simulink model "Final_V620140905h5b_fuben1"  (Simulink 7.9)
settings: Solver=FixedStepDiscrete  StartTime=0.0  StopTime=1  FixedStep=Auto  RelTol=1e-3
undefined symbols (not defined in the file or in its folder): Down, Up
libraries: tiiqmathlib x157, idelinklib_common x83, c2833xlib x37, simulink x12, c28xdmclib x12, c280xlib x7, simulink_extras x4, commutil2 x2, idelinklib_tgtpref x1, idelinklib_ticcs x1
(part 6 of 7)

== system Final_V620140905h5b_fuben1/Function-Call Subsystem1/AD/Read AD ==
  note: M2
  note: M1
  note: M12
  note: M11
  note: M9
  note: AD1
  note: AD2
  note: M10
  note: M3
  note: M4
  note: M5
  note: M6
  note: M7
  note: M8
  note: IH1
  note: IH3
  note: IH2
  note: IH4
  note: IH5
  note: VH1
  note: VH2
  note: VH9
  Memory Copy1 : idelinklib_common/Memory Copy  Priority=3  copyFrom=Specified address  copyFromAddressSource=Specify via dialog  copyFromAddress=hex2dec('200008')  copyFromSrcCode=myVariableSrc  dataTypeFrom=int16  dataDimensionFrom=1  useOffsetFrom=off  offsetFromSrc=Specify via dialog  offsetFrom=0  strideFrom=1  copyTo=Specified source code symbol  copyToAddressSource=Specify via dialog  copyToAddress=temp  copyToSrcCode=M8  dataTypeTo=int16  useOffsetTo=on  offsetToSrc=Specify via dialog  offsetTo=0  strideTo=1  sampleTime=inf  useInitValue=off  initValueSrc=Specify constant value  initValue=bin2dec('00000000')  initValueSrcCode=myInitValueVariable  useAsMask=off  maskOperator=bitwise AND  useTermValue=off  termValue=bin2dec('00000000')  isRealtimeEnabled=off  emitCCBeforeWrite=off  CCBeforeWrite=/* Custom Code Before Write*/  emitCCAfterWrite=off  CCAfterWrite=/* Custom Code After Write*/  useDMACopy=off  enableBlockingMode=off
  Memory Copy13 : idelinklib_common/Memory Copy  Priority=2  copyFrom=Specified address  copyFromAddressSource=Specify via dialog  copyFromAddress=hex2dec('200008')  copyFromSrcCode=myVariableSrc  dataTypeFrom=int16  dataDimensionFrom=1  useOffsetFrom=off  offsetFromSrc=Specify via dialog  offsetFrom=0  strideFrom=1  copyTo=Specified source code symbol  copyToAddressSource=Specify via dialog  copyToAddress=temp  copyToSrcCode=M7  dataTypeTo=int16  useOffsetTo=on  offsetToSrc=Specify via dialog  offsetTo=0  strideTo=1  sampleTime=inf  useInitValue=off  initValueSrc=Specify constant value  initValue=bin2dec('00000000')  initValueSrcCode=myInitValueVariable  useAsMask=off  maskOperator=bitwise AND  useTermValue=off  termValue=bin2dec('00000000')  isRealtimeEnabled=off  emitCCBeforeWrite=off  CCBeforeWrite=/* Custom Code Before Write*/  emitCCAfterWrite=off  CCAfterWrite=/* Custom Code After Write*/  useDMACopy=off  enableBlockingMode=off
  Memory Copy14 : idelinklib_common/Memory Copy  Priority=12  copyFrom=Specified address  copyFromAddressSource=Specify via dialog  copyFromAddress=hex2dec('200004')  copyFromSrcCode=myVariableSrc  dataTypeFrom=int16  dataDimensionFrom=1  useOffsetFrom=off  offsetFromSrc=Specify via dialog  offsetFrom=0  strideFrom=1  copyTo=Specified source code symbol  copyToAddressSource=Specify via dialog  copyToAddress=temp  copyToSrcCode=M4  dataTypeTo=int16  useOffsetTo=on  offsetToSrc=Specify via dialog  offsetTo=0  strideTo=1  sampleTime=inf  useInitValue=off  initValueSrc=Specify constant value  initValue=bin2dec('00000000')  initValueSrcCode=myInitValueVariable  useAsMask=off  maskOperator=bitwise AND  useTermValue=off  termValue=bin2dec('00000000')  isRealtimeEnabled=off  emitCCBeforeWrite=off  CCBeforeWrite=/* Custom Code Before Write*/  emitCCAfterWrite=off  CCAfterWrite=/* Custom Code After Write*/  useDMACopy=off  enableBlockingMode=off
  Memory Copy15 : idelinklib_common/Memory Copy  Priority=13  copyFrom=Specified address  copyFromAddressSource=Specify via dialog  copyFromAddress=hex2dec('200004')  copyFromSrcCode=myVariableSrc  dataTypeFrom=int16  dataDimensionFrom=1  useOffsetFrom=off  offsetFromSrc=Specify via dialog  offsetFrom=0  strideFrom=1  copyTo=Specified source code symbol  copyToAddressSource=Specify via dialog  copyToAddress=temp  copyToSrcCode=M5  dataTypeTo=int16  useOffsetTo=on  offsetToSrc=Specify via dialog  offsetTo=0  strideTo=1  sampleTime=inf  useInitValue=off  initValueSrc=Specify constant value  initValue=bin2dec('00000000')  initValueSrcCode=myInitValueVariable  useAsMask=off  maskOperator=bitwise AND  useTermValue=off  termValue=bin2dec('00000000')  isRealtimeEnabled=off  emitCCBeforeWrite=off  CCBeforeWrite=/* Custom Code Before Write*/  emitCCAfterWrite=off  CCAfterWrite=/* Custom Code After Write*/  useDMACopy=off  enableBlockingMode=off
  Memory Copy16 : idelinklib_common/Memory Copy  Priority=14  copyFrom=Specified address  copyFromAddressSource=Specify via dialog  copyFromAddress=hex2dec('200004')  copyFromSrcCode=myVariableSrc  dataTypeFrom=int16  dataDimensionFrom=1  useOffsetFrom=off  offsetFromSrc=Specify via dialog  offsetFrom=0  strideFrom=1  copyTo=Specified source code symbol  copyToAddressSource=Specify via dialog  copyToAddress=temp  copyToSrcCode=M6  dataTypeTo=int16  useOffsetTo=on  offsetToSrc=Specify via dialog  offsetTo=0  strideTo=1  sampleTime=inf  useInitValue=off  initValueSrc=Specify constant value  initValue=bin2dec('00000000')  initValueSrcCode=myInitValueVariable  useAsMask=off  maskOperator=bitwise AND  useTermValue=off  termValue=bin2dec('00000000')  isRealtimeEnabled=off  emitCCBeforeWrite=off  CCBeforeWrite=/* Custom Code Before Write*/  emitCCAfterWrite=off  CCAfterWrite=/* Custom Code After Write*/  useDMACopy=off  enableBlockingMode=off
  Memory Copy18 : idelinklib_common/Memory Copy  Priority=4  copyFrom=Specified address  copyFromAddressSource=Specify via dialog  copyFromAddress=hex2dec('200008')  copyFromSrcCode=myVariableSrc  dataTypeFrom=int16  dataDimensionFrom=1  useOffsetFrom=off  offsetFromSrc=Specify via dialog  offsetFrom=0  strideFrom=1  copyTo=Specified source code symbol  copyToAddressSource=Specify via dialog  copyToAddress=temp  copyToSrcCode=M9  dataTypeTo=int16  useOffsetTo=on  offsetToSrc=Specify via dialog  offsetTo=0  strideTo=1  sampleTime=inf  useInitValue=off  initValueSrc=Specify constant value  initValue=bin2dec('00000000')  initValueSrcCode=myInitValueVariable  useAsMask=off  maskOperator=bitwise AND  useTermValue=off  termValue=bin2dec('00000000')  isRealtimeEnabled=off  emitCCBeforeWrite=off  CCBeforeWrite=/* Custom Code Before Write*/  emitCCAfterWrite=off  CCAfterWrite=/* Custom Code After Write*/  useDMACopy=off  enableBlockingMode=off
  Memory Copy19 : idelinklib_common/Memory Copy  Priority=5  copyFrom=Specified address  copyFromAddressSource=Specify via dialog  copyFromAddress=hex2dec('200008')  copyFromSrcCode=myVariableSrc  dataTypeFrom=int16  dataDimensionFrom=1  useOffsetFrom=off  offsetFromSrc=Specify via dialog  offsetFrom=0  strideFrom=1  copyTo=Specified source code symbol  copyToAddressSource=Specify via dialog  copyToAddress=temp  copyToSrcCode=M10  dataTypeTo=int16  useOffsetTo=on  offsetToSrc=Specify via dialog  offsetTo=0  strideTo=1  sampleTime=inf  useInitValue=off  initValueSrc=Specify constant value  initValue=bin2dec('00000000')  initValueSrcCode=myInitValueVariable  useAsMask=off  maskOperator=bitwise AND  useTermValue=off  termValue=bin2dec('00000000')  isRealtimeEnabled=off  emitCCBeforeWrite=off  CCBeforeWrite=/* Custom Code Before Write*/  emitCCAfterWrite=off  CCAfterWrite=/* Custom Code After Write*/  useDMACopy=off  enableBlockingMode=off
  Memory Copy20 : idelinklib_common/Memory Copy  Priority=6  copyFrom=Specified address  copyFromAddressSource=Specify via dialog  copyFromAddress=hex2dec('200008')  copyFromSrcCode=myVariableSrc  dataTypeFrom=int16  dataDimensionFrom=1  useOffsetFrom=off  offsetFromSrc=Specify via dialog  offsetFrom=0  strideFrom=1  copyTo=Specified source code symbol  copyToAddressSource=Specify via dialog  copyToAddress=temp  copyToSrcCode=M11  dataTypeTo=int16  useOffsetTo=on  offsetToSrc=Specify via dialog  offsetTo=0  strideTo=1  sampleTime=inf  useInitValue=off  initValueSrc=Specify constant value  initValue=bin2dec('00000000')  initValueSrcCode=myInitValueVariable  useAsMask=off  maskOperator=bitwise AND  useTermValue=off  termValue=bin2dec('00000000')  isRealtimeEnabled=off  emitCCBeforeWrite=off  CCBeforeWrite=/* Custom Code Before Write*/  emitCCAfterWrite=off  CCAfterWrite=/* Custom Code After Write*/  useDMACopy=off  enableBlockingMode=off
  Memory Copy21 : idelinklib_common/Memory Copy  Priority=7  copyFrom=Specified address  copyFromAddressSource=Specify via dialog  copyFromAddress=hex2dec('200008')  copyFromSrcCode=myVariableSrc  dataTypeFrom=int16  dataDimensionFrom=1  useOffsetFrom=off  offsetFromSrc=Specify via dialog  offsetFrom=0  strideFrom=1  copyTo=Specified source code symbol  copyToAddressSource=Specify via dialog  copyToAddress=temp  copyToSrcCode=M12  dataTypeTo=int16  useOffsetTo=on  offsetToSrc=Specify via dialog  offsetTo=0  strideTo=1  sampleTime=inf  useInitValue=off  initValueSrc=Specify constant value  initValue=bin2dec('00000000')  initValueSrcCode=myInitValueVariable  useAsMask=off  maskOperator=bitwise AND  useTermValue=off  termValue=bin2dec('00000000')  isRealtimeEnabled=off  emitCCBeforeWrite=off  CCBeforeWrite=/* Custom Code Before Write*/  emitCCAfterWrite=off  CCAfterWrite=/* Custom Code After Write*/  useDMACopy=off  enableBlockingMode=off
  Memory Copy22 : idelinklib_common/Memory Copy  Priority=9  copyFrom=Specified address  copyFromAddressSource=Specify via dialog  copyFromAddress=hex2dec('200004')  copyFromSrcCode=myVariableSrc  dataTypeFrom=int16  dataDimensionFrom=1  useOffsetFrom=off  offsetFromSrc=Specify via dialog  offsetFrom=0  strideFrom=1  copyTo=Specified source code symbol  copyToAddressSource=Specify via dialog  copyToAddress=temp  copyToSrcCode=M1  dataTypeTo=int16  useOffsetTo=on  offsetToSrc=Specify via dialog  offsetTo=0  strideTo=1  sampleTime=inf  useInitValue=off  initValueSrc=Specify constant value  initValue=bin2dec('00000000')  initValueSrcCode=myInitValueVariable  useAsMask=off  maskOperator=bitwise AND  useTermValue=off  termValue=bin2dec('00000000')  isRealtimeEnabled=off  emitCCBeforeWrite=off  CCBeforeWrite=/* Custom Code Before Write*/  emitCCAfterWrite=off  CCAfterWrite=/* Custom Code After Write*/  useDMACopy=off  enableBlockingMode=off
  Memory Copy23 : idelinklib_common/Memory Copy  Priority=10  copyFrom=Specified address  copyFromAddressSource=Specify via dialog  copyFromAddress=hex2dec('200004')  copyFromSrcCode=myVariableSrc  dataTypeFrom=int16  dataDimensionFrom=1  useOffsetFrom=off  offsetFromSrc=Specify via dialog  offsetFrom=0  strideFrom=1  copyTo=Specified source code symbol  copyToAddressSource=Specify via dialog  copyToAddress=temp  copyToSrcCode=M2  dataTypeTo=int16  useOffsetTo=on  offsetToSrc=Specify via dialog  offsetTo=0  strideTo=1  sampleTime=inf  useInitValue=off  initValueSrc=Specify constant value  initValue=bin2dec('00000000')  initValueSrcCode=myInitValueVariable  useAsMask=off  maskOperator=bitwise AND  useTermValue=off  termValue=bin2dec('00000000')  isRealtimeEnabled=off  emitCCBeforeWrite=off  CCBeforeWrite=/* Custom Code Before Write*/  emitCCAfterWrite=off  CCAfterWrite=/* Custom Code After Write*/  useDMACopy=off  enableBlockingMode=off
  Memory Copy24 : idelinklib_common/Memory Copy  Priority=11  copyFrom=Specified address  copyFromAddressSource=Specify via dialog  copyFromAddress=hex2dec('200004')  copyFromSrcCode=myVariableSrc  dataTypeFrom=int16  dataDimensionFrom=1  useOffsetFrom=off  offsetFromSrc=Specify via dialog  offsetFrom=0  strideFrom=1  copyTo=Specified source code symbol  copyToAddressSource=Specify via dialog  copyToAddress=temp  copyToSrcCode=M3  dataTypeTo=int16  useOffsetTo=on  offsetToSrc=Specify via dialog  offsetTo=0  strideTo=1  sampleTime=inf  useInitValue=off  initValueSrc=Specify constant value  initValue=bin2dec('00000000')  initValueSrcCode=myInitValueVariable  useAsMask=off  maskOperator=bitwise AND  useTermValue=off  termValue=bin2dec('00000000')  isRealtimeEnabled=off  emitCCBeforeWrite=off  CCBeforeWrite=/* Custom Code Before Write*/  emitCCAfterWrite=off  CCAfterWrite=/* Custom Code After Write*/  useDMACopy=off  enableBlockingMode=off

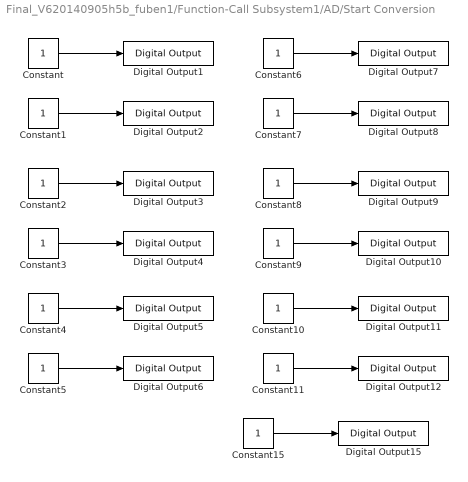
== system Final_V620140905h5b_fuben1/Function-Call Subsystem1/AD/Start Conversion ==
  Constant{,1..11,15} (13 alike) : Constant  OutDataTypeStr=boolean
  Digital Output{1,3..12,15} (12 alike) : c2833xlib/Digital Output  Priority=1  GPIO_Number=GPIO56~GPIO63  GPIO_Bit0=off  GPIO_BIT0_Toggle=off  GPIO_Bit1=on  GPIO_BIT1_Toggle=off  GPIO_Bit2=off  GPIO_BIT2_Toggle=off  GPIO_Bit3=off  GPIO_BIT3_Toggle=off  GPIO_Bit4=off  GPIO_BIT4_Toggle=off  GPIO_Bit5=off  GPIO_BIT5_Toggle=off  GPIO_Bit6=off  GPIO_BIT6_Toggle=off  GPIO_Bit7=off  GPIO_BIT7_Toggle=off
  Digital Output2 : c2833xlib/Digital Output  Priority=1  GPIO_Number=GPIO56~GPIO63  GPIO_Bit0=off  GPIO_BIT0_Toggle=off  GPIO_Bit1=off  GPIO_BIT1_Toggle=off  GPIO_Bit2=on  GPIO_BIT2_Toggle=off  GPIO_Bit3=off  GPIO_BIT3_Toggle=off  GPIO_Bit4=off  GPIO_BIT4_Toggle=off  GPIO_Bit5=off  GPIO_BIT5_Toggle=off  GPIO_Bit6=off  GPIO_BIT6_Toggle=off  GPIO_Bit7=off  GPIO_BIT7_Toggle=off
  wires:
  Constant/1 -> Digital Output1/1
  Constant1/1 -> Digital Output2/1
  Constant2/1 -> Digital Output3/1
  Constant3/1 -> Digital Output4/1
  Constant4/1 -> Digital Output5/1
  Constant5/1 -> Digital Output6/1
  Constant6/1 -> Digital Output7/1
  Constant7/1 -> Digital Output8/1
  Constant8/1 -> Digital Output9/1
  Constant9/1 -> Digital Output10/1
  Constant10/1 -> Digital Output11/1
  Constant11/1 -> Digital Output12/1
  Constant15/1 -> Digital Output15/1

== system Final_V620140905h5b_fuben1/Function-Call Subsystem1/AD/Stop Conversion ==
  Constant12 : Constant  Value=0  OutDataTypeStr=boolean
  Constant14 : Constant  Value=0  OutDataTypeStr=boolean
  Digital Output13 : c2833xlib/Digital Output  Priority=8  GPIO_Number=GPIO56~GPIO63  GPIO_Bit0=off  GPIO_BIT0_Toggle=off  GPIO_Bit1=on  GPIO_BIT1_Toggle=off  GPIO_Bit2=off  GPIO_BIT2_Toggle=off  GPIO_Bit3=off  GPIO_BIT3_Toggle=off  GPIO_Bit4=off  GPIO_BIT4_Toggle=off  GPIO_Bit5=off  GPIO_BIT5_Toggle=off  GPIO_Bit6=off  GPIO_BIT6_Toggle=off  GPIO_Bit7=off  GPIO_BIT7_Toggle=off
  Digital Output14 : c2833xlib/Digital Output  Priority=15  GPIO_Number=GPIO56~GPIO63  GPIO_Bit0=off  GPIO_BIT0_Toggle=off  GPIO_Bit1=off  GPIO_BIT1_Toggle=off  GPIO_Bit2=on  GPIO_BIT2_Toggle=off  GPIO_Bit3=off  GPIO_BIT3_Toggle=off  GPIO_Bit4=off  GPIO_BIT4_Toggle=off  GPIO_Bit5=off  GPIO_BIT5_Toggle=off  GPIO_Bit6=off  GPIO_BIT6_Toggle=off  GPIO_Bit7=off  GPIO_BIT7_Toggle=off
  wires:
  Constant12/1 -> Digital Output13/1
  Constant14/1 -> Digital Output14/1

== system Final_V620140905h5b_fuben1/Function-Call Subsystem1/Nr measure/ION multiply1 ==
  x : Inport
  Constant2 : Constant  Value=x  OutDataTypeStr=Inherit: Inherit via back propagation
  IQN x IQN : tiiqmathlib/IQN x IQN  multiplyOption=Multiply
  Kx : Outport
  wires:
  IQN x IQN/1 -> Kx/1
  x/1 -> IQN x IQN/1
  Constant2/1 -> IQN x IQN/2

== system Final_V620140905h5b_fuben1/Function-Call Subsystem1/Nr measure/ION multiply18 ==
  x : Inport
  Constant2 : Constant  Value=x  OutDataTypeStr=Inherit: Inherit via back propagation
  IQN x IQN : tiiqmathlib/IQN x IQN  multiplyOption=Multiply
  Kx : Outport
  wires:
  Constant2/1 -> IQN x IQN/2
  x/1 -> IQN x IQN/1
  IQN x IQN/1 -> Kx/1

== system Final_V620140905h5b_fuben1/Function-Call Subsystem1/Nr measure/Integration 0 to maximal3 ==
  x : Inport
  3 : Constant  Value=a  OutDataTypeStr=fixdt(1,32,16)
  Relational Operator1 : RelationalOperator  Operator=<=
  Sum1 : Sum  Inputs=+-
  Sum2 : Sum
  Switch2 : Switch  Criteria=u2 > Threshold  SaturateOnIntegerOverflow=on  InputSameDT=on
  Unit Delay1 : UnitDelay  SampleTime=-1
  y : Outport
  Zero Trig : Outport  Port=2
  wires:
  x/1 -> Sum2/2
  Sum1/1 -> Switch2/3
  Switch2/1 -> y/1, Unit Delay1/1
  Relational Operator1/1 -> Zero Trig/1, Switch2/2
  3/1 -> Sum1/2, Relational Operator1/2
  Sum2/1 -> Sum1/1, Relational Operator1/1, Switch2/1
  Unit Delay1/1 -> Sum2/1

== system Final_V620140905h5b_fuben1/Function-Call Subsystem1/Nr measure/Triggered Subsystem1 ==
  Trigger : TriggerPort  TriggerType=falling
  Sum10 : Sum  Inputs=+-
  Unit Delay5 : UnitDelay  SampleTime=-1
  eQEP : c280xlib/eQEP  useModule=eQEP2  pcInputmode=Up-count  externalClockrate=1x resolution: Count the rising edge only  swapPolarityselection=Clockwise  qdfOutputport=off  qapPolarityselection=off  qbpPolarityselection=off  qipPolarityselection=off  qspPolarityselection=off  igatePolarityselection=off  sampleTime=-1  pcOutputport=on  pcMaximumvalue=1024  indexInitializationcheck=off  indexInitializationevent=Rising edge  strobeInitializationcheck=off  strobeInitializationevent=Rising edge  softwareInitializationcheck=off  softwareInitializationsource=Set to init value at start up  softwareInitializationmode=on  pcInitialvalue=0  pcResetmode=Reset on the maximum position  ieloutputport=off  indexEventlatch=Rising edge  seloutputport=off  strobeEventlatch=Rising edge  pcefOutputport=off  enableEqepcapture=off  qctmrOutputport=off  qcprdOutputport=off  captureTimerprescaler=128  upEventprescaler=128  overflowErrorflag=off  directionErrorflag=off  captureTimerposition=On position counter read  unitTimerperiod=100000000  captureTimerlatch=off  capturePeriodlatch=off  positionCounterlatch=off  soenPolarityselection=off  spselPolarityselection=Index pin is used for sync output  compareValuesource=Specify via dialog  shadowMode=Load on QPOSCNT=0  compareValue=4294967295  syncOutputwidth=1  polaritySyncoutput=Active high  watchdogEnable=off  watchdogTimer=65535  outport1Datatype=auto  outport2Datatype=int16  outport3Datatype=auto  outport4Datatype=auto  outport5Datatype=auto  outport6Datatype=auto  outport7Datatype=auto  outport8Datatype=auto  outport9Datatype=auto  outport10Datatype=auto  outport11Datatype=auto  outport12Datatype=auto  eqepinterrupt_pce=off  eqepinterrupt_qpe=off  eqepinterrupt_qdc=off  eqepinterrupt_wto=off  eqepinterrupt_pcu=off  eqepinterrupt_pco=off  eqepinterrupt_pcr=off  eqepinterrupt_pcm=off  eqepinterrupt_sel=off  eqepinterrupt_iel=off  eqepinterrupt_uto=off  pheOutputport=off  watchdogOutputport=off  outport13Datatype=auto  outport14Datatype=auto
  Out1 : Outport
  wires:
  Unit Delay5/1 -> Sum10/2
  Sum10/1 -> Out1/1
  eQEP/1 -> Sum10/1, Unit Delay5/1

== system Final_V620140905h5b_fuben1/Function-Call Subsystem1/Nr protect/ION multiply2 ==
  x : Inport
  Constant2 : Constant  Value=x  OutDataTypeStr=fixdt(1,32,16)
  IQN x IQN : tiiqmathlib/IQN x IQN  multiplyOption=Multiply
  Kx : Outport
  wires:
  IQN x IQN/1 -> Kx/1
  x/1 -> IQN x IQN/1
  Constant2/1 -> IQN x IQN/2

== system Final_V620140905h5b_fuben1/Function-Call Subsystem1/Nr protect/ION multiply3 ==
  x : Inport
  Constant2 : Constant  Value=x  OutDataTypeStr=fixdt(1,32,16)
  IQN x IQN : tiiqmathlib/IQN x IQN  multiplyOption=Multiply
  Kx : Outport
  wires:
  IQN x IQN/1 -> Kx/1
  x/1 -> IQN x IQN/1
  Constant2/1 -> IQN x IQN/2

== system Final_V620140905h5b_fuben1/Function-Call Subsystem1/Nr protect/Triggered Subsystem1 ==
  Reset1 : Inport
  Trigger : TriggerPort  TriggerType=falling
  Constant12 : Constant  OutDataTypeStr=fixdt(1,32,16)
  Counter1 : Subsystem
  Count1 : Outport
  wires:
  Constant12/1 -> Counter1/1(x)
  Reset1/1 -> Counter1/2(Reset)
  Counter1/1(y) -> Count1/1

== system Final_V620140905h5b_fuben1/Function-Call Subsystem1/Nr protect/sample per n times ==
  x : Inport
  Absolute IQN : tiiqmathlib/Absolute IQN
  Constant12 : Constant  OutDataTypeStr=fixdt(1,32,16)
  Constant13 : Constant  Value=n  OutDataTypeStr=fixdt(1,32,16)
  Counter1 : Subsystem
  Counter2 : Subsystem
  Relational Operator2 : RelationalOperator
  Triggered Subsystem1 : Subsystem  TreatAsAtomicUnit=on
  Unit Delay2 : UnitDelay  SampleTime=-1
  sum : Outport
  wires:
  Absolute IQN/1 -> Counter2/1(x)
  Constant12/1 -> Counter1/1(x)
  Counter1/1(y) -> Relational Operator2/2
  Constant13/1 -> Relational Operator2/1
  Relational Operator2/1 -> Unit Delay2/1, Triggered Subsystem1/Trigger
  Unit Delay2/1 -> Counter1/2(Reset), Counter2/2(Reset)
  Counter2/1(y) -> Triggered Subsystem1/1(in)
  x/1 -> Absolute IQN/1
  Triggered Subsystem1/1(out) -> sum/1

== system Final_V620140905h5b_fuben1/Function-Call Subsystem1/PI-1/RC filter1 ==
  x : Inport
  Constant2 : Constant  Value=a  OutDataTypeStr=fixdt(1,32,16)
  Constant3 : Constant  Value=1-a  OutDataTypeStr=fixdt(1,32,16)
  IQN x IQN : tiiqmathlib/IQN x IQN  multiplyOption=Multiply
  IQN x IQN1 : tiiqmathlib/IQN x IQN  multiplyOption=Multiply
  Sum2 : Sum
  Unit Delay2 : UnitDelay  SampleTime=-1
  y : Outport
  wires:
  x/1 -> IQN x IQN/1
  Constant2/1 -> IQN x IQN/2
  Constant3/1 -> IQN x IQN1/1
  IQN x IQN/1 -> Sum2/1
  IQN x IQN1/1 -> Sum2/2
  Sum2/1 -> y/1, Unit Delay2/1
  Unit Delay2/1 -> IQN x IQN1/2

== system Final_V620140905h5b_fuben1/Function-Call Subsystem1/PI-3/RC filter1 ==
  x : Inport
  Constant2 : Constant  Value=a  OutDataTypeStr=fixdt(1,32,16)
  Constant3 : Constant  Value=1-a  OutDataTypeStr=fixdt(1,32,16)
  IQN x IQN : tiiqmathlib/IQN x IQN  multiplyOption=Multiply
  IQN x IQN1 : tiiqmathlib/IQN x IQN  multiplyOption=Multiply
  Sum2 : Sum
  Unit Delay2 : UnitDelay  SampleTime=-1
  y : Outport
  wires:
  x/1 -> IQN x IQN/1
  Constant2/1 -> IQN x IQN/2
  Constant3/1 -> IQN x IQN1/1
  IQN x IQN/1 -> Sum2/1
  IQN x IQN1/1 -> Sum2/2
  Sum2/1 -> y/1, Unit Delay2/1
  Unit Delay2/1 -> IQN x IQN1/2

== system Final_V620140905h5b_fuben1/Function-Call Subsystem1/PI-4/RC filter1 ==
  x : Inport
  Constant2 : Constant  Value=a  OutDataTypeStr=fixdt(1,32,16)
  Constant3 : Constant  Value=1-a  OutDataTypeStr=fixdt(1,32,16)
  IQN x IQN : tiiqmathlib/IQN x IQN  multiplyOption=Multiply
  IQN x IQN1 : tiiqmathlib/IQN x IQN  multiplyOption=Multiply
  Sum2 : Sum
  Unit Delay2 : UnitDelay  SampleTime=-1
  y : Outport
  wires:
  Unit Delay2/1 -> IQN x IQN1/2
  Sum2/1 -> Unit Delay2/1, y/1
  IQN x IQN1/1 -> Sum2/2
  IQN x IQN/1 -> Sum2/1
  Constant3/1 -> IQN x IQN1/1
  Constant2/1 -> IQN x IQN/2
  x/1 -> IQN x IQN/1

== system Final_V620140905h5b_fuben1/Function-Call Subsystem1/PI-5/RC filter1 ==
  x : Inport
  Constant2 : Constant  Value=a  OutDataTypeStr=fixdt(1,32,16)
  Constant3 : Constant  Value=1-a  OutDataTypeStr=fixdt(1,32,16)
  IQN x IQN : tiiqmathlib/IQN x IQN  multiplyOption=Multiply
  IQN x IQN1 : tiiqmathlib/IQN x IQN  multiplyOption=Multiply
  Sum2 : Sum
  Unit Delay2 : UnitDelay  SampleTime=-1
  y : Outport
  wires:
  Unit Delay2/1 -> IQN x IQN1/2
  Sum2/1 -> Unit Delay2/1, y/1
  IQN x IQN1/1 -> Sum2/2
  IQN x IQN/1 -> Sum2/1
  Constant3/1 -> IQN x IQN1/1
  Constant2/1 -> IQN x IQN/2
  x/1 -> IQN x IQN/1

== system Final_V620140905h5b_fuben1/Function-Call Subsystem1/Soft-start1/Integration 0 to maximal1 ==
  x : Inport
  Reset : Inport  Port=2
  Constant1 : Constant  Value=0  OutDataTypeStr=fixdt(1,32,16)
  Saturation1 : Saturate  UpperLimit=b  LowerLimit=0  LinearizeAsGain=off  ZeroCross=off  OutDataTypeStr=fixdt(1,32,16)
  Sum2 : Sum
  Switch2 : Switch  Criteria=u2 > Threshold  SaturateOnIntegerOverflow=on  InputSameDT=on
  Unit Delay1 : UnitDelay  SampleTime=-1
  y : Outport
  wires:
  Saturation1/1 -> y/1, Unit Delay1/1
  Reset/1 -> Switch2/2
  Constant1/1 -> Switch2/3
  x/1 -> Sum2/2
  Switch2/1 -> Saturation1/1
  Sum2/1 -> Switch2/1
  Unit Delay1/1 -> Sum2/1

== system Final_V620140905h5b_fuben1/Function-Call Subsystem1/Soft-start2/Integration 0 to maximal1 ==
  x : Inport
  Reset : Inport  Port=2
  Constant1 : Constant  Value=0  OutDataTypeStr=fixdt(1,32,16)
  Saturation1 : Saturate  UpperLimit=b  LowerLimit=0  LinearizeAsGain=off  ZeroCross=off  OutDataTypeStr=fixdt(1,32,16)
  Sum2 : Sum
  Switch2 : Switch  Criteria=u2 > Threshold  SaturateOnIntegerOverflow=on  InputSameDT=on
  Unit Delay1 : UnitDelay  SampleTime=-1
  y : Outport
  wires:
  Unit Delay1/1 -> Sum2/1
  Sum2/1 -> Switch2/1
  Switch2/1 -> Saturation1/1
  x/1 -> Sum2/2
  Constant1/1 -> Switch2/3
  Reset/1 -> Switch2/2
  Saturation1/1 -> Unit Delay1/1, y/1

== system Final_V620140905h5b_fuben1/Function-Call Subsystem1/Soft-start4/Integration 0 to maximal1 ==
  x : Inport
  Reset : Inport  Port=2
  Constant1 : Constant  Value=0  OutDataTypeStr=fixdt(1,32,16)
  Saturation1 : Saturate  UpperLimit=1  LowerLimit=0  LinearizeAsGain=off  ZeroCross=off  OutDataTypeStr=fixdt(1,32,16)
  Sum2 : Sum
  Switch2 : Switch  Criteria=u2 > Threshold  SaturateOnIntegerOverflow=on  InputSameDT=on
  Unit Delay1 : UnitDelay  SampleTime=-1
  y : Outport
  wires:
  Saturation1/1 -> y/1, Unit Delay1/1
  Reset/1 -> Switch2/2
  Constant1/1 -> Switch2/3
  x/1 -> Sum2/2
  Switch2/1 -> Saturation1/1
  Sum2/1 -> Switch2/1
  Unit Delay1/1 -> Sum2/1

== system Final_V620140905h5b_fuben1/Function-Call Subsystem1/Soft-start5/Integration 0 to maximal1 ==
  x : Inport
  Reset : Inport  Port=2
  Constant1 : Constant  Value=0  OutDataTypeStr=fixdt(1,32,16)
  Saturation1 : Saturate  UpperLimit=b  LowerLimit=0  LinearizeAsGain=off  ZeroCross=off  OutDataTypeStr=fixdt(1,32,16)
  Sum2 : Sum
  Switch2 : Switch  Criteria=u2 > Threshold  SaturateOnIntegerOverflow=on  InputSameDT=on
  Unit Delay1 : UnitDelay  SampleTime=-1
  y : Outport
  wires:
  Saturation1/1 -> y/1, Unit Delay1/1
  Reset/1 -> Switch2/2
  Constant1/1 -> Switch2/3
  x/1 -> Sum2/2
  Switch2/1 -> Saturation1/1
  Sum2/1 -> Switch2/1
  Unit Delay1/1 -> Sum2/1

== system Final_V620140905h5b_fuben1/Function-Call Subsystem1/Soft-start6/Integration 0 to maximal1 ==
  x : Inport
  Reset : Inport  Port=2
  Constant1 : Constant  Value=0  OutDataTypeStr=fixdt(1,32,16)
  Saturation1 : Saturate  UpperLimit=b  LowerLimit=0  LinearizeAsGain=off  ZeroCross=off  OutDataTypeStr=fixdt(1,32,16)
  Sum2 : Sum
  Switch2 : Switch  Criteria=u2 > Threshold  SaturateOnIntegerOverflow=on  InputSameDT=on
  Unit Delay1 : UnitDelay  SampleTime=-1
  y : Outport
  wires:
  Saturation1/1 -> y/1, Unit Delay1/1
  Reset/1 -> Switch2/2
  Constant1/1 -> Switch2/3
  x/1 -> Sum2/2
  Switch2/1 -> Saturation1/1
  Sum2/1 -> Switch2/1
  Unit Delay1/1 -> Sum2/1

== system Final_V620140905h5b_fuben1/Function-Call Subsystem1/Soft_turn_on/Voltage soft start (from 0 to 1 within 10s)1 ==
  Reset : Inport
  Constant1 : Constant  Value=0  OutDataTypeStr=fixdt(1,32,16)
  Constant29 : Constant  Value=0.02*(b-c)/a  OutDataTypeStr=fixdt(1,32,16)
  ION multiply1 : Subsystem  mask{x=1/100}
      mask prompts: x "gain"
  Saturation1 : Saturate  UpperLimit=b*100  LowerLimit=c*100  LinearizeAsGain=off  ZeroCross=off  OutDataTypeStr=fixdt(1,32,16)
  Sum2 : Sum
  Switch2 : Switch  Criteria=u2 > Threshold  SaturateOnIntegerOverflow=on  InputSameDT=on
  Unit Delay1 : UnitDelay  SampleTime=-1
  k : Outport
  wires:
  Unit Delay1/1 -> Sum2/1
  Sum2/1 -> Switch2/1
  Switch2/1 -> Saturation1/1
  Constant29/1 -> Sum2/2
  Constant1/1 -> Switch2/3
  Reset/1 -> Switch2/2
  Saturation1/1 -> Unit Delay1/1, ION multiply1/1(x)
  ION multiply1/1(Kx) -> k/1

== system Final_V620140905h5b_fuben1/Function-Call Subsystem1/Soft_turn_on/Voltage soft start (from 0 to 120 within 5s) ==
  Reset : Inport
  Constant1 : Constant  Value=0  OutDataTypeStr=fixdt(1,32,16)
  Constant29 : Constant  Value=0.02*(b-c)/a  OutDataTypeStr=fixdt(1,32,16)
  ION multiply1 : Subsystem  mask{x=1/100}
      mask prompts: x "gain"
  Saturation1 : Saturate  UpperLimit=b*100  LowerLimit=c*100  LinearizeAsGain=off  ZeroCross=off  OutDataTypeStr=fixdt(1,32,16)
  Sum2 : Sum
  Switch2 : Switch  Criteria=u2 > Threshold  SaturateOnIntegerOverflow=on  InputSameDT=on
  Unit Delay1 : UnitDelay  SampleTime=-1
  k : Outport
  wires:
  ION multiply1/1(Kx) -> k/1
  Saturation1/1 -> ION multiply1/1(x), Unit Delay1/1
  Reset/1 -> Switch2/2
  Constant1/1 -> Switch2/3
  Constant29/1 -> Sum2/2
  Switch2/1 -> Saturation1/1
  Sum2/1 -> Switch2/1
  Unit Delay1/1 -> Sum2/1

== system Final_V620140905h5b_fuben1/Function-Call Subsystem1/Subsystem/Triggered Subsystem1 ==
  Reset1 : Inport
  Trigger : TriggerPort  TriggerType=falling
  Constant12 : Constant  OutDataTypeStr=fixdt(1,32,16)
  Counter1 : Subsystem
  Count1 : Outport
  wires:
  Constant12/1 -> Counter1/1(x)
  Reset1/1 -> Counter1/2(Reset)
  Counter1/1(y) -> Count1/1

== system Final_V620140905h5b_fuben1/Function-Call Subsystem1/Subsystem/sample per n times ==
  x : Inport
  Absolute IQN : tiiqmathlib/Absolute IQN
  Constant12 : Constant  OutDataTypeStr=fixdt(1,32,16)
  Constant13 : Constant  Value=n  OutDataTypeStr=fixdt(1,32,16)
  Counter1 : Subsystem
  Counter2 : Subsystem
  Relational Operator2 : RelationalOperator
  Triggered Subsystem1 : Subsystem  TreatAsAtomicUnit=on
  Unit Delay2 : UnitDelay  SampleTime=-1
  sum : Outport
  wires:
  Absolute IQN/1 -> Counter2/1(x)
  Constant12/1 -> Counter1/1(x)
  Counter1/1(y) -> Relational Operator2/2
  Constant13/1 -> Relational Operator2/1
  Relational Operator2/1 -> Unit Delay2/1, Triggered Subsystem1/Trigger
  Unit Delay2/1 -> Counter1/2(Reset), Counter2/2(Reset)
  Counter2/1(y) -> Triggered Subsystem1/1(in)
  x/1 -> Absolute IQN/1
  Triggered Subsystem1/1(out) -> sum/1

== system Final_V620140905h5b_fuben1/Function-Call Subsystem1/Subsystem1/ION multiply1 ==
  x : Inport
  Constant2 : Constant  Value=x  OutDataTypeStr=fixdt(1,32,16)
  IQN x IQN : tiiqmathlib/IQN x IQN  multiplyOption=Multiply
  Kx : Outport
  wires:
  Constant2/1 -> IQN x IQN/2
  x/1 -> IQN x IQN/1
  IQN x IQN/1 -> Kx/1

== system Final_V620140905h5b_fuben1/Function-Call Subsystem1/Subsystem1/ION multiply16 ==
  x : Inport
  Constant2 : Constant  Value=x  OutDataTypeStr=fixdt(1,32,16)
  IQN x IQN : tiiqmathlib/IQN x IQN  multiplyOption=Multiply
  Kx : Outport
  wires:
  IQN x IQN/1 -> Kx/1
  x/1 -> IQN x IQN/1
  Constant2/1 -> IQN x IQN/2

== system Final_V620140905h5b_fuben1/Function-Call Subsystem1/Subsystem1/ION multiply17 ==
  x : Inport
  Constant2 : Constant  Value=x  OutDataTypeStr=fixdt(1,32,16)
  IQN x IQN : tiiqmathlib/IQN x IQN  multiplyOption=Multiply
  Kx : Outport
  wires:
  Constant2/1 -> IQN x IQN/2
  x/1 -> IQN x IQN/1
  IQN x IQN/1 -> Kx/1

== system Final_V620140905h5b_fuben1/Function-Call Subsystem1/Voltage protect/RC filter11 ==
  x : Inport
  Constant2 : Constant  Value=a  OutDataTypeStr=fixdt(1,32,16)
  Constant3 : Constant  Value=1-a  OutDataTypeStr=fixdt(1,32,16)
  IQN x IQN : tiiqmathlib/IQN x IQN  multiplyOption=Multiply
  IQN x IQN1 : tiiqmathlib/IQN x IQN  multiplyOption=Multiply
  Sum2 : Sum
  Unit Delay2 : UnitDelay  SampleTime=-1
  y : Outport
  wires:
  Unit Delay2/1 -> IQN x IQN1/2
  Sum2/1 -> Unit Delay2/1, y/1
  IQN x IQN1/1 -> Sum2/2
  IQN x IQN/1 -> Sum2/1
  Constant3/1 -> IQN x IQN1/1
  Constant2/1 -> IQN x IQN/2
  x/1 -> IQN x IQN/1

== system Final_V620140905h5b_fuben1/Function-Call Subsystem1/abc/dq-grid voltage1/RC filter1 ==
  x : Inport
  Constant2 : Constant  Value=a  OutDataTypeStr=fixdt(1,32,16)
  Constant3 : Constant  Value=1-a  OutDataTypeStr=fixdt(1,32,16)
  IQN x IQN : tiiqmathlib/IQN x IQN  multiplyOption=Multiply
  IQN x IQN1 : tiiqmathlib/IQN x IQN  multiplyOption=Multiply
  Sum2 : Sum
  Unit Delay2 : UnitDelay  SampleTime=-1
  y : Outport
  wires:
  Unit Delay2/1 -> IQN x IQN1/2
  Sum2/1 -> Unit Delay2/1, y/1
  IQN x IQN1/1 -> Sum2/2
  IQN x IQN/1 -> Sum2/1
  Constant3/1 -> IQN x IQN1/1
  Constant2/1 -> IQN x IQN/2
  x/1 -> IQN x IQN/1

== system Final_V620140905h5b_fuben1/Function-Call Subsystem1/abc/dq-grid voltage1/RC filter5 ==
  x : Inport
  Constant2 : Constant  Value=a  OutDataTypeStr=fixdt(1,32,16)
  Constant3 : Constant  Value=1-a  OutDataTypeStr=fixdt(1,32,16)
  IQN x IQN : tiiqmathlib/IQN x IQN  multiplyOption=Multiply
  IQN x IQN1 : tiiqmathlib/IQN x IQN  multiplyOption=Multiply
  Sum2 : Sum
  Unit Delay2 : UnitDelay  SampleTime=-1
  y : Outport
  wires:
  x/1 -> IQN x IQN/1
  Constant2/1 -> IQN x IQN/2
  Constant3/1 -> IQN x IQN1/1
  IQN x IQN/1 -> Sum2/1
  IQN x IQN1/1 -> Sum2/2
  Sum2/1 -> y/1, Unit Delay2/1
  Unit Delay2/1 -> IQN x IQN1/2

== system Final_V620140905h5b_fuben1/Function-Call Subsystem1/abc/dq-grid voltage5/ION multiply17 ==
  x : Inport
  Constant2 : Constant  Value=x  OutDataTypeStr=fixdt(1,32,16)
  IQN x IQN : tiiqmathlib/IQN x IQN  multiplyOption=Multiply
  Kx : Outport
  wires:
  IQN x IQN/1 -> Kx/1
  x/1 -> IQN x IQN/1
  Constant2/1 -> IQN x IQN/2

== system Final_V620140905h5b_fuben1/Function-Call Subsystem1/abc/dq-grid voltage7/RC filter1 ==
  x : Inport
  Constant2 : Constant  Value=a  OutDataTypeStr=fixdt(1,32,16)
  Constant3 : Constant  Value=1-a  OutDataTypeStr=fixdt(1,32,16)
  IQN x IQN : tiiqmathlib/IQN x IQN  multiplyOption=Multiply
  IQN x IQN1 : tiiqmathlib/IQN x IQN  multiplyOption=Multiply
  Sum2 : Sum
  Unit Delay2 : UnitDelay  SampleTime=-1
  y : Outport
  wires:
  x/1 -> IQN x IQN/1
  Constant2/1 -> IQN x IQN/2
  Constant3/1 -> IQN x IQN1/1
  IQN x IQN/1 -> Sum2/1
  IQN x IQN1/1 -> Sum2/2
  Sum2/1 -> y/1, Unit Delay2/1
  Unit Delay2/1 -> IQN x IQN1/2

== system Final_V620140905h5b_fuben1/Function-Call Subsystem1/abc/dq-grid voltage7/RC filter5 ==
  x : Inport
  Constant2 : Constant  Value=a  OutDataTypeStr=fixdt(1,32,16)
  Constant3 : Constant  Value=1-a  OutDataTypeStr=fixdt(1,32,16)
  IQN x IQN : tiiqmathlib/IQN x IQN  multiplyOption=Multiply
  IQN x IQN1 : tiiqmathlib/IQN x IQN  multiplyOption=Multiply
  Sum2 : Sum
  Unit Delay2 : UnitDelay  SampleTime=-1
  y : Outport
  wires:
  Unit Delay2/1 -> IQN x IQN1/2
  Sum2/1 -> Unit Delay2/1, y/1
  IQN x IQN1/1 -> Sum2/2
  IQN x IQN/1 -> Sum2/1
  Constant3/1 -> IQN x IQN1/1
  Constant2/1 -> IQN x IQN/2
  x/1 -> IQN x IQN/1

== system Final_V620140905h5b_fuben1/Function-Call Subsystem1/set and reset/Soft-start3 ==
  Reset : Inport
  Constant29 : Constant  Value=a  OutDataTypeStr=fixdt(1,32,16)
  Integration 0 to maximal1 : Subsystem
  Vref : Outport
  wires:
  Constant29/1 -> Integration 0 to maximal1/1(x)
  Integration 0 to maximal1/1(y) -> Vref/1
  Reset/1 -> Integration 0 to maximal1/2(Reset)

== system Final_V620140905h5b_fuben1/Function-Call Subsystem1/Nr protect/Triggered Subsystem1/Counter1 ==
  x : Inport
  Reset : Inport  Port=2
  Constant11 : Constant  Value=0  OutDataTypeStr=fixdt(1,32,16)
  Saturation : Saturate  UpperLimit=1000  LowerLimit=0  LinearizeAsGain=off  ZeroCross=off  OutDataTypeStr=fixdt(1,32,16)
  Sum2 : Sum
  Switch2 : Switch  Criteria=u2 > Threshold  SaturateOnIntegerOverflow=on  InputSameDT=on
  Unit Delay1 : UnitDelay  SampleTime=-1
  y : Outport
  wires:
  Saturation/1 -> Unit Delay1/1, y/1
  Constant11/1 -> Switch2/3
  x/1 -> Sum2/2
  Switch2/1 -> Saturation/1
  Reset/1 -> Switch2/2
  Sum2/1 -> Switch2/1
  Unit Delay1/1 -> Sum2/1

== system Final_V620140905h5b_fuben1/Function-Call Subsystem1/Nr protect/sample per n times/Counter1 ==
  x : Inport
  Reset : Inport  Port=2
  Constant11 : Constant  Value=0  OutDataTypeStr=fixdt(1,32,16)
  Saturation : Saturate  UpperLimit=10000  LowerLimit=0  LinearizeAsGain=off  ZeroCross=off  OutDataTypeStr=fixdt(1,32,16)
  Sum2 : Sum
  Switch2 : Switch  Criteria=u2 > Threshold  SaturateOnIntegerOverflow=on  InputSameDT=on
  Unit Delay1 : UnitDelay  SampleTime=-1
  y : Outport
  wires:
  Saturation/1 -> Unit Delay1/1, y/1
  Constant11/1 -> Switch2/3
  x/1 -> Sum2/2
  Switch2/1 -> Saturation/1
  Reset/1 -> Switch2/2
  Sum2/1 -> Switch2/1
  Unit Delay1/1 -> Sum2/1

== system Final_V620140905h5b_fuben1/Function-Call Subsystem1/Nr protect/sample per n times/Counter2 ==
  x : Inport
  Reset : Inport  Port=2
  Constant11 : Constant  Value=0  OutDataTypeStr=fixdt(1,32,16)
  Saturation : Saturate  UpperLimit=10000  LowerLimit=0  LinearizeAsGain=off  ZeroCross=off  OutDataTypeStr=fixdt(1,32,16)
  Sum2 : Sum
  Switch2 : Switch  Criteria=u2 > Threshold  SaturateOnIntegerOverflow=on  InputSameDT=on
  Unit Delay1 : UnitDelay  SampleTime=-1
  y : Outport
  wires:
  Unit Delay1/1 -> Sum2/1
  Sum2/1 -> Switch2/1
  Reset/1 -> Switch2/2
  Switch2/1 -> Saturation/1
  x/1 -> Sum2/2
  Constant11/1 -> Switch2/3
  Saturation/1 -> y/1, Unit Delay1/1

== system Final_V620140905h5b_fuben1/Function-Call Subsystem1/Nr protect/sample per n times/Triggered Subsystem1 ==
  in : Inport
  Trigger : TriggerPort  TriggerType=falling
  out : Outport
  wires:
  in/1 -> out/1

== system Final_V620140905h5b_fuben1/Function-Call Subsystem1/Soft_turn_on/Voltage soft start (from 0 to 1 within 10s)1/ION multiply1 ==
  x : Inport
  Constant2 : Constant  Value=x  OutDataTypeStr=fixdt(1,32,16)
  IQN x IQN : tiiqmathlib/IQN x IQN  multiplyOption=Multiply
  Kx : Outport
  wires:
  IQN x IQN/1 -> Kx/1
  x/1 -> IQN x IQN/1
  Constant2/1 -> IQN x IQN/2

== system Final_V620140905h5b_fuben1/Function-Call Subsystem1/Soft_turn_on/Voltage soft start (from 0 to 120 within 5s)/ION multiply1 ==
  x : Inport
  Constant2 : Constant  Value=x  OutDataTypeStr=fixdt(1,32,16)
  IQN x IQN : tiiqmathlib/IQN x IQN  multiplyOption=Multiply
  Kx : Outport
  wires:
  Constant2/1 -> IQN x IQN/2
  x/1 -> IQN x IQN/1
  IQN x IQN/1 -> Kx/1

== system Final_V620140905h5b_fuben1/Function-Call Subsystem1/Subsystem/Triggered Subsystem1/Counter1 ==
  x : Inport
  Reset : Inport  Port=2
  Constant11 : Constant  Value=0  OutDataTypeStr=fixdt(1,32,16)
  Saturation : Saturate  UpperLimit=10000  LowerLimit=0  LinearizeAsGain=off  ZeroCross=off  OutDataTypeStr=fixdt(1,32,16)
  Sum2 : Sum
  Switch2 : Switch  Criteria=u2 > Threshold  SaturateOnIntegerOverflow=on  InputSameDT=on
  Unit Delay1 : UnitDelay  SampleTime=-1
  y : Outport
  wires:
  Saturation/1 -> Unit Delay1/1, y/1
  Constant11/1 -> Switch2/3
  x/1 -> Sum2/2
  Switch2/1 -> Saturation/1
  Reset/1 -> Switch2/2
  Sum2/1 -> Switch2/1
  Unit Delay1/1 -> Sum2/1

== system Final_V620140905h5b_fuben1/Function-Call Subsystem1/Subsystem/sample per n times/Counter1 ==
  x : Inport
  Reset : Inport  Port=2
  Constant11 : Constant  Value=0  OutDataTypeStr=fixdt(1,32,16)
  Saturation : Saturate  UpperLimit=10000  LowerLimit=0  LinearizeAsGain=off  ZeroCross=off  OutDataTypeStr=fixdt(1,32,16)
  Sum2 : Sum
  Switch2 : Switch  Criteria=u2 > Threshold  SaturateOnIntegerOverflow=on  InputSameDT=on
  Unit Delay1 : UnitDelay  SampleTime=-1
  y : Outport
  wires:
  Saturation/1 -> Unit Delay1/1, y/1
  Constant11/1 -> Switch2/3
  x/1 -> Sum2/2
  Switch2/1 -> Saturation/1
  Reset/1 -> Switch2/2
  Sum2/1 -> Switch2/1
  Unit Delay1/1 -> Sum2/1

== system Final_V620140905h5b_fuben1/Function-Call Subsystem1/Subsystem/sample per n times/Counter2 ==
  x : Inport
  Reset : Inport  Port=2
  Constant11 : Constant  Value=0  OutDataTypeStr=fixdt(1,32,16)
  Saturation : Saturate  UpperLimit=10000  LowerLimit=0  LinearizeAsGain=off  ZeroCross=off  OutDataTypeStr=fixdt(1,32,16)
  Sum2 : Sum
  Switch2 : Switch  Criteria=u2 > Threshold  SaturateOnIntegerOverflow=on  InputSameDT=on
  Unit Delay1 : UnitDelay  SampleTime=-1
  y : Outport
  wires:
  Unit Delay1/1 -> Sum2/1
  Sum2/1 -> Switch2/1
  Reset/1 -> Switch2/2
  Switch2/1 -> Saturation/1
  x/1 -> Sum2/2
  Constant11/1 -> Switch2/3
  Saturation/1 -> y/1, Unit Delay1/1

== system Final_V620140905h5b_fuben1/Function-Call Subsystem1/Subsystem/sample per n times/Triggered Subsystem1 ==
  in : Inport
  Trigger : TriggerPort  TriggerType=falling
  out : Outport
  wires:
  in/1 -> out/1

== system Final_V620140905h5b_fuben1/Function-Call Subsystem1/set and reset/Soft-start3/Integration 0 to maximal1 ==
  x : Inport
  Reset : Inport  Port=2
  Constant1 : Constant  Value=0  OutDataTypeStr=fixdt(1,32,16)
  Saturation1 : Saturate  UpperLimit=b  LowerLimit=0  LinearizeAsGain=off  ZeroCross=off  OutDataTypeStr=fixdt(1,32,16)
  Sum2 : Sum
  Switch2 : Switch  Criteria=u2 > Threshold  SaturateOnIntegerOverflow=on  InputSameDT=on
  Unit Delay1 : UnitDelay  SampleTime=-1
  y : Outport
  wires:
  Unit Delay1/1 -> Sum2/1
  Sum2/1 -> Switch2/1
  Switch2/1 -> Saturation1/1
  x/1 -> Sum2/2
  Constant1/1 -> Switch2/3
  Reset/1 -> Switch2/2
  Saturation1/1 -> Unit Delay1/1, y/1

== stateflow chart Control Logic ==
  state Close
    during: State=0;
  state Track_Voltage_NoPll_Vgrid
    during: State=1;
  state Phase_Locking_Vgrid_Pll
    during: State=2;
  state Grid_Connecting
    during: State=3;
  state Alone_Generating_Vg_Nopll_G1orG2_Disconnected
    during: State=4;
  state False
    during: State=10;
  state Alone_Generating_Vg_pll_G1orG2_Disconnecting
    during: State=5;
  state Alone_Generating_Vgrid_Nopll
    during: State=6;
  state Alone_Generating_Vgrid_Pll
    during: State=7;
  state Alone_Generating_Vg_pll_G_Disconnecting
    during: State=9;
  state Alone_Generating_G_Disconnecting_Waiting
    during: State=8;
  state G1orG2_Connecting_Waiting
    during: State=11;
  state Alone_Generating_Vg_NoPll
    during: State=12;
  (default) -> Close
  Close -> Track_Voltage_NoPll_Vgrid [order 1] : [On==0&&Vbus==1]
  Track_Voltage_NoPll_Vgrid -> Close [order 3] : [On==1&&KM==0]
  Track_Voltage_NoPll_Vgrid -> Phase_Locking_Vgrid_Pll [order 1] : [Vs==1&&On==0]
  Phase_Locking_Vgrid_Pll -> Grid_Connecting [order 2] : [PLL==1&&On==0]
  Alone_Generating_Vgrid_Nopll -> Alone_Generating_Vgrid_Pll [order 1] : [On==0&&Vs==1]
  Alone_Generating_Vg_Nopll_G1orG2_Disconnected -> False [order 1] : [Fault==1]
  Alone_Generating_Vg_NoPll -> Track_Voltage_NoPll_Vgrid [order 3] : [On==0&&Vbus==1]
  Track_Voltage_NoPll_Vgrid -> False [order 2] : [Fault==1]
  Phase_Locking_Vgrid_Pll -> False [order 1] : [Fault==1]
  Grid_Connecting -> False [order 3] : [Fault==1]
  Phase_Locking_Vgrid_Pll -> Track_Voltage_NoPll_Vgrid [order 3] : [On==1]
  Close -> Alone_Generating_Vg_Nopll_G1orG2_Disconnected [order 2] : [On==0&&Vbus==0]
  Alone_Generating_Vg_Nopll_G1orG2_Disconnected -> Close [order 2] : [On==1]
  Grid_Connecting -> Track_Voltage_NoPll_Vgrid [order 1] : [On==1]
  Alone_Generating_Vgrid_Pll -> G1orG2_Connecting_Waiting [order 1] : [On==0&&PLL==1]
  Grid_Connecting -> Alone_Generating_Vg_pll_G1orG2_Disconnecting [order 2] : [On==0&&Sg==1&&Vbus==1]
  False -> Close : [On==1]
  Alone_Generating_Vg_pll_G1orG2_Disconnecting -> False [order 1] : [Fault==1]
  Alone_Generating_Vg_pll_G1orG2_Disconnecting -> Alone_Generating_Vg_Nopll_G1orG2_Disconnected [order 2] : [On==0&&Vg1==0&&Vg2==0]
  Alone_Generating_Vg_Nopll_G1orG2_Disconnected -> Alone_Generating_Vgrid_Nopll [order 3] : [On==0&&Vg2==1]
  Alone_Generating_Vg_pll_G1orG2_Disconnecting -> Close [order 3] : [On==1]
  Alone_Generating_G_Disconnecting_Waiting -> Close [order 3] : [On==1]
  Alone_Generating_Vg_Nopll_G1orG2_Disconnected -> Alone_Generating_Vgrid_Nopll [order 4] : [On==0&&Vg1==1]
  Alone_Generating_Vg_pll_G_Disconnecting -> Close [order 1] : [On==1]
  Alone_Generating_Vgrid_Nopll -> False [order 2] : [Fault==1]
  G1orG2_Connecting_Waiting -> Alone_Generating_G_Disconnecting_Waiting [order 1] : [On==0&&S_G1==1]
  Alone_Generating_G_Disconnecting_Waiting -> False [order 1] : [Fault==1]
  Alone_Generating_Vg_pll_G_Disconnecting -> False [order 2] : [Fault==1]
  Alone_Generating_Vgrid_Nopll -> Close [order 3] : [On==1]
  Alone_Generating_Vgrid_Pll -> Close [order 2] : [On==1]
  Alone_Generating_Vgrid_Pll -> False [order 3] : [Fault==1]
  G1orG2_Connecting_Waiting -> False [order 2] : [Fault==1]
  G1orG2_Connecting_Waiting -> Close [order 3] : [On==1]
  Alone_Generating_Vg_pll_G_Disconnecting -> Alone_Generating_Vg_NoPll [order 3] : [On==0&&Vg1==0&&Vg2==0]
  Alone_Generating_Vg_NoPll -> Close [order 1] : [On==1]
  Alone_Generating_Vg_NoPll -> False [order 2] : [Fault==1]
  Alone_Generating_G_Disconnecting_Waiting -> Alone_Generating_Vg_pll_G_Disconnecting [order 2] : [On==0&&Sg1==1]
  data: State output uint16; Vbus input uint16; Fault input uint16; On input uint16; Vs input uint16; KM input uint16; PLL input uint16; Sg input uint16; Vg1 input uint16; Vg2 input uint16; S_G1 input uint16; Sg1 input uint16

== stateflow chart Control Logic1 ==
  state State1
    during:
  state State2
    entry: K1=K1+0.2;
  state State0
    entry: K1=3; K2=0.015; K3=2.5;
  state State3
    entry: K1=K1-0.2;
  state State4
    entry: K2=K2+0.002;
  state State5
    entry: K2=K2-0.002;
  state State6
    entry: K3=K3+0.1;
  state State7
    entry: K3=K3-0.1;
  (default) -> State0
  State1 -> State2 [order 5] : [Ch==3&&Inc==0]
  State2 -> State1 : [Inc==1]
  State0 -> State1
  State1 -> State3 [order 1] : [Ch==3&&Dec==0]
  State3 -> State1 : [Dec==1]
  State1 -> State4 [order 6] : [Ch==4&&Inc==0]
  State4 -> State1 : [Inc==1]
  State1 -> State5 [order 3] : [Ch==4&&Dec==0]
  State5 -> State1 : [Dec==1]
  State1 -> State6 [order 4] : [Ch==5&&Inc==0]
  State6 -> State1 : [Inc==1]
  State1 -> State7 [order 2] : [Ch==5&&Dec==0]
  State7 -> State1 : [Dec==1]
  data: Ch input uint16; Inc input uint16; Dec input uint16; K1 output fixdt(1,32,16); K2 output fixdt(1,32,16); K3 output fixdt(1,32,16)

== stateflow chart Control Logic2 ==
  state State1
    during: K=0;
  state State6
    during: K=0;
  state State3
    entry: Out=Out+1;
  state State4
    entry: Out=0;
  State6 -> State1 : [In==1]
  State1 -> State3 : [In==0]
  State3 -> State6 [order 2] : [Out<=26]
  (default) -> State1
  State4 -> State6
  State3 -> State4 [order 1] : [Out>26]
  data: In input uint16; Out output uint16; K local uint16

== stateflow chart Control Logic3 ==
  state State1
    during:
  state State2
    entry: K1=K1+0.02;
  state State0
    entry: K1=0.1; K2=0.0033; K3=0.6;
  state State3
    entry: K1=K1-0.02;
  state State4
    entry: K2=K2+0.0002;
  state State5
    entry: K2=K2-0.0002;
  state State6
    entry: K3=K3+0.1;
  state State7
    entry: K3=K3-0.1;
  (default) -> State0
  State1 -> State2 [order 5] : [Ch==0&&Inc==0]
  State2 -> State1 : [Inc==1]
  State0 -> State1
  State1 -> State3 [order 1] : [Ch==0&&Dec==0]
  State3 -> State1 : [Dec==1]
  State1 -> State4 [order 6] : [Ch==1&&Inc==0]
  State4 -> State1 : [Inc==1]
  State1 -> State5 [order 3] : [Ch==1&&Dec==0]
  State5 -> State1 : [Dec==1]
  State1 -> State6 [order 4] : [Ch==2&&Inc==0]
  State6 -> State1 : [Inc==1]
  State1 -> State7 [order 2] : [Ch==2&&Dec==0]
  State7 -> State1 : [Dec==1]
  data: Ch input uint16; Inc input uint16; Dec input uint16; K1 output fixdt(1,32,16); K2 output fixdt(1,32,16); K3 output fixdt(1,32,16)

== stateflow chart Control Logic4 ==
  state State1
    during:
  state State2
    entry: K1=K1+1;
  state State0
    entry: K1=20; K2=30; K3=20;
  state State3
    entry: K1=K1-1;
  state State4
    entry: K2=K2+1;
  state State5
    entry: K2=K2-1;
  state State6
    entry: K3=K3+1;
  state State7
    entry: K3=K3-1;
  (default) -> State0
  State1 -> State2 [order 5] : [Ch==6&&Inc==0]
  State2 -> State1 : [Inc==1]
  State0 -> State1
  State1 -> State3 [order 1] : [Ch==6&&Dec==0]
  State3 -> State1 : [Dec==1]
  State1 -> State4 [order 6] : [Ch==7&&Inc==0]
  State4 -> State1 : [Inc==1]
  State1 -> State5 [order 3] : [Ch==7&&Dec==0]
  State5 -> State1 : [Dec==1]
  State1 -> State6 [order 4] : [Ch==8&&Inc==0]
  State6 -> State1 : [Inc==1]
  State1 -> State7 [order 2] : [Ch==8&&Dec==0]
  State7 -> State1 : [Dec==1]
  data: Ch input uint16; Inc input uint16; Dec input uint16; K1 output fixdt(1,32,16); K2 output fixdt(1,32,16); K3 output fixdt(1,32,16)

== stateflow chart Control Logic5 ==
  state State1
    during:
  state State2
    entry: K1=K1+0.02;
  state State0
    entry: K1=0.21; K2=0.019; K3=1.3;
  state State3
    entry: K1=K1-0.02;
  state State4
    entry: K2=K2+0.002;
  state State5
    entry: K2=K2-0.002;
  state State6
    entry: K3=K3+0.1;
  state State7
    entry: K3=K3-0.1;
  (default) -> State0
  State1 -> State2 [order 5] : [Ch==9&&Inc==0]
  State2 -> State1 : [Inc==1]
  State0 -> State1
  State1 -> State3 [order 1] : [Ch==9&&Dec==0]
  State3 -> State1 : [Dec==1]
  State1 -> State4 [order 6] : [Ch==10&&Inc==0]
  State4 -> State1 : [Inc==1]
  State1 -> State5 [order 3] : [Ch==10&&Dec==0]
  State5 -> State1 : [Dec==1]
  State1 -> State6 [order 4] : [Ch==11&&Inc==0]
  State6 -> State1 : [Inc==1]
  State1 -> State7 [order 2] : [Ch==11&&Dec==0]
  State7 -> State1 : [Dec==1]
  data: Ch input uint16; Inc input uint16; Dec input uint16; K1 output fixdt(1,32,16); K2 output fixdt(1,32,16); K3 output fixdt(1,32,16)

== stateflow chart Control Logic6 ==
  state State1
    during:
  state State2
    entry: K1=K1+1;
  state State0
    entry: K1=15; K2=15; K3=100;
  state State3
    entry: K1=K1-1;
  state State4
    entry: K2=K2+1;
  state State5
    entry: K2=K2-1;
  state State6
    entry: K3=K3+1;
  state State7
    entry: K3=K3-1;
  (default) -> State0
  State1 -> State2 [order 5] : [Ch==12&&Inc==0]
  State2 -> State1 : [Inc==1]
  State0 -> State1
  State1 -> State3 [order 1] : [Ch==12&&Dec==0]
  State3 -> State1 : [Dec==1]
  State1 -> State4 [order 6] : [Ch==13&&Inc==0]
  State4 -> State1 : [Inc==1]
  State1 -> State5 [order 3] : [Ch==13&&Dec==0]
  State5 -> State1 : [Dec==1]
  State1 -> State6 [order 4] : [Ch==14&&Inc==0]
  State6 -> State1 : [Inc==1]
  State1 -> State7 [order 2] : [Ch==14&&Dec==0]
  State7 -> State1 : [Dec==1]
  data: Ch input uint16; Inc input uint16; Dec input uint16; K1 output fixdt(1,32,16); K2 output fixdt(1,32,16); K3 output fixdt(1,32,16)

== stateflow chart Control Logic7 ==
  state State1
    during:
  state State2
    entry: K1=K1+0.02;
  state State0
    entry: K1=0.25; K2=0; K3=0.6;
  state State3
    entry: K1=K1-0.02;
  state State4
    entry: K2=K2+0.02;
  state State5
    entry: K2=K2-0.02;
  state State6
    entry: K3=K3+0.1;
  state State7
    entry: K3=K3-0.1;
  (default) -> State0
  State1 -> State2 [order 5] : [Ch==15&&Inc==0]
  State2 -> State1 : [Inc==1]
  State0 -> State1
  State1 -> State3 [order 1] : [Ch==15&&Dec==0]
  State3 -> State1 : [Dec==1]
  State1 -> State4 [order 6] : [Ch==16&&Inc==0]
  State4 -> State1 : [Inc==1]
  State1 -> State5 [order 3] : [Ch==16&&Dec==0]
  State5 -> State1 : [Dec==1]
  State1 -> State6 [order 4] : [Ch==17&&Inc==0]
  State6 -> State1 : [Inc==1]
  State1 -> State7 [order 2] : [Ch==17&&Dec==0]
  State7 -> State1 : [Dec==1]
  data: Ch input uint16; Inc input uint16; Dec input uint16; K1 output fixdt(1,32,16); K2 output fixdt(1,32,16); K3 output fixdt(1,32,16)

== stateflow chart Control Logic8 ==
  state State1
    during:
  state State2
    entry: K1=K1+1;
  state State0
    entry: K1=55; K2=50; K3=50;
  state State3
    entry: K1=K1-1;
  state State4
    entry: K2=K2+1;
  state State5
    entry: K2=K2-1;
  state State6
    entry: K3=K3+1;
  state State7
    entry: K3=K3-1;
  (default) -> State0
  State1 -> State2 [order 5] : [Ch==18&&Inc==0]
  State2 -> State1 : [Inc==1]
  State0 -> State1
  State1 -> State3 [order 1] : [Ch==18&&Dec==0]
  State3 -> State1 : [Dec==1]
  State1 -> State4 [order 6] : [Ch==19&&Inc==0]
  State4 -> State1 : [Inc==1]
  State1 -> State5 [order 3] : [Ch==19&&Dec==0]
  State5 -> State1 : [Dec==1]
  State1 -> State6 [order 4] : [Ch==20&&Inc==0]
  State6 -> State1 : [Inc==1]
  State1 -> State7 [order 2] : [Ch==20&&Dec==0]
  State7 -> State1 : [Dec==1]
  data: Ch input uint16; Inc input uint16; Dec input uint16; K1 output fixdt(1,32,16); K2 output fixdt(1,32,16); K3 output fixdt(1,32,16)

== stateflow chart Control Logic9 ==
  state State1
    during:
  state State2
    entry: K1=K1+0.01;
  state State0
    entry: K1=0.29; K2=0.013; K3=0.3;
  state State3
    entry: K1=K1-0.01;
  state State4
    entry: K2=K2+0.002;
  state State5
    entry: K2=K2-0.002;
  state State6
    entry: K3=K3+0.1;
  state State7
    entry: K3=K3-0.1;
  (default) -> State0
  State1 -> State2 [order 5] : [Ch==21&&Inc==0]
  State2 -> State1 : [Inc==1]
  State0 -> State1
  State1 -> State3 [order 1] : [Ch==21&&Dec==0]
  State3 -> State1 : [Dec==1]
  State1 -> State4 [order 6] : [Ch==22&&Inc==0]
  State4 -> State1 : [Inc==1]
  State1 -> State5 [order 3] : [Ch==22&&Dec==0]
  State5 -> State1 : [Dec==1]
  State1 -> State6 [order 4] : [Ch==23&&Inc==0]
  State6 -> State1 : [Inc==1]
  State1 -> State7 [order 2] : [Ch==23&&Dec==0]
  State7 -> State1 : [Dec==1]
  data: Ch input uint16; Inc input uint16; Dec input uint16; K1 output fixdt(1,32,16); K2 output fixdt(1,32,16); K3 output fixdt(1,32,16)

== stateflow chart Control Logic10 ==
  state State1
    during:
  state State2
    entry: K1=K1+0.02;
  state State0
    entry: K1=0.2; K2=0.01; K3=4;
  state State3
    entry: K1=K1-0.02;
  state State4
    entry: K2=K2+0.02;
  state State5
    entry: K2=K2-0.02;
  state State6
    entry: K3=K3+0.01;
  state State7
    entry: K3=K3-0.01;
  (default) -> State0
  State1 -> State2 [order 5] : [Ch==24&&Inc==0]
  State2 -> State1 : [Inc==1]
  State0 -> State1
  State1 -> State3 [order 1] : [Ch==24&&Dec==0]
  State3 -> State1 : [Dec==1]
  State1 -> State4 [order 6] : [Ch==25&&Inc==0]
  State4 -> State1 : [Inc==1]
  State1 -> State5 [order 3] : [Ch==25&&Dec==0]
  State5 -> State1 : [Dec==1]
  State1 -> State6 [order 4] : [Ch==26&&Inc==0]
  State6 -> State1 : [Inc==1]
  State1 -> State7 [order 2] : [Ch==26&&Dec==0]
  State7 -> State1 : [Dec==1]
  data: Ch input uint16; Inc input uint16; Dec input uint16; K1 output fixdt(1,32,16); K2 output fixdt(1,32,16); K3 output fixdt(1,32,16)
